simulink model "Rod_end_v7c"  (R2023a)
settings: Solver=ode1be  StartTime=0.0  StopTime=3  FixedStep=1e-6  MaxStep=1e-5  RelTol=1e-3
values from neighbouring files (symbols this model uses):
  A1_la = 5.710000e-003    (= 0.00571)    [C1_Actuator_1_Data.m]
  A2_la = 5.710000e-003    (= 0.00571)    [C1_Actuator_1_Data.m]
  a_jetpipe_area = 0    [B2_Main_file_Double_Active_Standby_System.m]
  A_svfb = 79.12.*1E-9.*sqrt(pi)    [B2_Main_file_Double_Active_Standby_System.m]
  a_svfb0_1 = 1E-3    (= 0.001)    [B2_Main_file_Double_Active_Standby_System.m]
  a_svfb0_2 = 0    [B2_Main_file_Double_Active_Standby_System.m]
  Afl_sv = dfl_sv^2*pi/4    (= 2.01519637574e-09)    [C1_Actuator_1_Data.m]
  Ag_sv = 18e-6    (= 1.8e-05)    [C1_Actuator_1_Data.m]
  air_gap0_1 = 0    [B2_Main_file_Double_Active_Standby_System.m]
  air_gap_fault_time = 10000    [B2_Main_file_Double_Active_Standby_System.m]
  Alpha_p0 = eta-acos((L^2+t^2-s^2)/(2*L*t))    [Parametri_rod_end.m]
  Asp_sv = 1.35e-5    (= 1.35e-05)    [C1_Actuator_1_Data.m]
  B0_sv = 0.460    (= 0.46)    [C1_Actuator_1_Data.m]
  b_airgap = 0.3    [B2_Main_file_Double_Active_Standby_System.m]
  b_fbspring = 2E-3    (= 0.002)    [B2_Main_file_Double_Active_Standby_System.m]
  b_max = 0*0.0001    (= 0)    [C1_Actuator_1_Data.m]
  beta = 800000000    [D4_Fluid.m]    (also in Rapporto_di_trasmissione.m = acos((L-t.*cos(alpha))./s))
  Beta0 = acos((L-t*cos(Alpha0))/s)    [Parametri_rod_end.m]
  beta_LVDT = 0    [aggiunte.m]
  bf_sv = 0.45    [C1_Actuator_1_Data.m]
  bsp_sv = 0.25    [C1_Actuator_1_Data.m]
  c = 55    [Parametri_rod_end.m]
  C_svfb = 1    [B2_Main_file_Double_Active_Standby_System.m]
  Cdmax_sv = 0.7392    [C1_Actuator_1_Data.m]
  Cdmin_sv = 0.6428    [C1_Actuator_1_Data.m]
  CLa = 900000    [aggiunte.m]
  Csa_la = 0.02*sqrt(Ksa_la*Meq_la)    [C1_Actuator_1_Data.m]
  Damping = 1e3    (= 1000)    [Parametri_rod_end.m]
  Damping_rot = 100    [Parametri_rod_end.m]
  Del_on = 1    [B2_Main_file_Double_Active_Standby_System.m]
  demag0_1 = 0    [B2_Main_file_Double_Active_Standby_System.m]
  dfl_sv = 5.0654e-5    (= 5.0654e-05)    [C1_Actuator_1_Data.m]
  dt_sim = 1e-5    (= 1e-05)    [B2_Main_file_Double_Active_Standby_System.m]
  enable_jetpipe_distorsion = 0    [B2_Main_file_Double_Active_Standby_System.m]
  eta = deg2rad(15)    [Parametri_rod_end.m]
  F_att_sv = 4    [C1_Actuator_1_Data.m]
  FH = FH+0.175*pi*Dd_se(ii)*(-0.884+0.0206*Hs_se(ii)-0.0001*(Hs_se(ii))^2)*Tw_se(ii)    [D2_Data_seal.m]
  first_cycle = 0    [B2_Main_file_Double_Active_Standby_System.m]
  flight_hours = 8    [B2_Main_file_Double_Active_Standby_System.m]
  g = 9.81    [Parametri_rod_end.m]
  g_sv = G_sv/l0_sv    (= 0)    [C1_Actuator_1_Data.m]
  Gamma_la = 1.667e4    (= 16670)    [C1_Actuator_1_Data.m]
  gap_ms = 0    [C1_Actuator_1_Data.m]
  Gq_sv = 0.069    [C1_Actuator_1_Data.m]
  Gust_stiffness_jetpipe = 1e8    (= 100000000)    [B2_Main_file_Double_Active_Standby_System.m]
  Gust_threshold = 10000    [B2_Main_file_Double_Active_Standby_System.m]
  h_fbspring = 1E-3    (= 0.001)    [B2_Main_file_Double_Active_Standby_System.m]
  h_sv = H_sv/l0_sv    (= 0)    [C1_Actuator_1_Data.m]
  hr_sv = 6e-6    (= 6e-06)    [C1_Actuator_1_Data.m]
  hyd_fluid_repl = 20    [B2_Main_file_Double_Active_Standby_System.m]
  I = 2.3    [Parametri_rod_end.m]    (also in Rapporto_di_trasmissione.m)
  imax_sv = 8e-3    (= 0.008)    [C1_Actuator_1_Data.m]
  Initial_condition = [0;0;0.000]    [Parametri_rod_end.m]
  Ixx_out = 0.0000321    (= 3.21e-05)    [Parametri_rod_end.m]
  Iyy_in = 0.0000008    (= 8e-07)    [Parametri_rod_end.m]
  Iyy_out = 0.0000035    (= 3.5e-06)    [Parametri_rod_end.m]
  Izz_in = 0.00000011    (= 1.1e-07)    [Parametri_rod_end.m]
  Izz_out = 0.0000337    (= 3.37e-05)    [Parametri_rod_end.m]
  Ja_sv = 1.0575e-5    (= 1.0575e-05)    [C1_Actuator_1_Data.m]
  jetpipe_initialpos = 0    [B2_Main_file_Double_Active_Standby_System.m]
  jetpipe_passage_area = 1    [B2_Main_file_Double_Active_Standby_System.m]
  k = 4/(3*pi*(sigma_j+sigma_k))*((R_in*R_out)/(R_in+R_out))^0.5    (= 15092124693.8)    [Parametri_rod_end.m]
  k_airgap = 0.5/100*0.01    (= 5e-05)    [B2_Main_file_Double_Active_Standby_System.m]
  k_c0_jetpipe_area = 0*1e-1    (= 0)    [B2_Main_file_Double_Active_Standby_System.m]
  k_sv = mup_sv*Vp_sv/(2*B0_sv*l0_sv)-1    (= 16.0383594613)    [C1_Actuator_1_Data.m]
  Kf_sv = 301.6    [C1_Actuator_1_Data.m]
  KFPi = zeros(m,1)    [D2_Data_seal.m]
  Kli1 = 0    [C1_Actuator_1_Data.m]
  Kli2 = 0    [C1_Actuator_1_Data.m]
  Ksa_la = 12480000    [C1_Actuator_1_Data.m]
  Kw_sv = 14.5    [C1_Actuator_1_Data.m]
  L = 0.37    [Parametri_rod_end.m]    (also in Rapporto_di_trasmissione.m = l+delta_l)
  l0_sv = 0.5e-3    (= 0.0005)    [C1_Actuator_1_Data.m]
  L_c = imax_sv    (= 0.008)    [C1_Actuator_1_Data.m]
  L_la1 = 0.059900    (= 0.0599)    [C1_Actuator_1_Data.m]
  L_la2 = 0.084800    (= 0.0848)    [C1_Actuator_1_Data.m]
  la_sv = 41e-3    (= 0.041)    [C1_Actuator_1_Data.m]
  lambda_LVDT = 0*0.005*1.5    (= 0)    [aggiunte.m]
  lf = 0.025    [C1_Actuator_1_Data.m]    (also in C2_Actuator_2_Data.m)
  LVDTsize0 = 1    [aggiunte.m]
  m_in = 0.0215    [Parametri_rod_end.m]
  m_out = 0.1    [Parametri_rod_end.m]
  m_thermal = 0    [B2_Main_file_Double_Active_Standby_System.m]
  Mcyl_la = 30.425550    (= 30.42555)    [C1_Actuator_1_Data.m]
  Mrod_la = 11.313490    (= 11.31349)    [C1_Actuator_1_Data.m]
  msp_sv = 0.005    [C1_Actuator_1_Data.m]
  mua_sv = 4*pi/1e7    (= 1.25663706144e-06)    [C1_Actuator_1_Data.m]
  mup_sv = 1.1*4*pi/1e7    (= 1.38230076758e-06)    [C1_Actuator_1_Data.m]
  n1_sv = 1140    [C1_Actuator_1_Data.m]
  n2_sv = 1140    [C1_Actuator_1_Data.m]
  n_svfb = 3    [B2_Main_file_Double_Active_Standby_System.m]
  null_shift = -1+2*rand(1,1)    [B2_Main_file_Double_Active_Standby_System.m]
  null_shift_sign = -1+((-1+2*rand(1,1))>=0)*2    [B2_Main_file_Double_Active_Standby_System.m]
  OV_R1 = 0*2.344e-05    (= 0)    [C1_Actuator_1_Data.m]
  OV_R2 = 0*2.344e-05    (= 0)    [C1_Actuator_1_Data.m]
  OV_S1 = 0*2.344e-05    (= 0)    [C1_Actuator_1_Data.m]
  OV_S2 = 0*2.344e-05    (= 0)    [C1_Actuator_1_Data.m]
  P01_la = Pmean-DP_eq    [C1_Actuator_1_Data.m]
  P02_la = Pmean+DP_eq    [C1_Actuator_1_Data.m]
  perc_passage_area0_1 = 0    [B2_Main_file_Double_Active_Standby_System.m]
  Pocl_A = 0    [C1_Actuator_1_Data.m]
  Pocl_B = 0    [C1_Actuator_1_Data.m]
  Pr = 600000    [B2_Main_file_Double_Active_Standby_System.m]
  Ps = 35000000    [B2_Main_file_Double_Active_Standby_System.m]
  R_in = 0.019    [Parametri_rod_end.m]
  R_out = 0.0195    [Parametri_rod_end.m]
  R_th1 = 0    [B2_Main_file_Double_Active_Standby_System.m]
  Remax_sv = 5000    [C1_Actuator_1_Data.m]
  Resistance = 1    [C1_Actuator_1_Data.m]
  rj_sv = 1e-6    (= 1e-06)    [C1_Actuator_1_Data.m]
  Rp02_svspring = 1014    [B2_Main_file_Double_Active_Standby_System.m]
  s = 0.11    [Parametri_rod_end.m]    (also in Rapporto_di_trasmissione.m)
  sigma_0LVDT = 0*0.01*1.5*5    (= 0)    [aggiunte.m]
  ST_AD = ceil(10000/fs_AD)/10000    [C1_Actuator_1_Data.m]
  Stiffness_rot = 1e3    (= 1000)    [Parametri_rod_end.m]
  Stifness = 1e8    (= 100000000)    [Parametri_rod_end.m]
  sv_crackON1 = 0    [B2_Main_file_Double_Active_Standby_System.m]
  sv_crackON2 = 0    [B2_Main_file_Double_Active_Standby_System.m]
  T0 = 0    [aggiunte.m]
  tau_w1 = 0    [B2_Main_file_Double_Active_Standby_System.m]
  ... (+14 more)
undefined symbols (not defined in the file or in its folder): Ixx_in, magnitude, mass, muu, Newton, R_sp_C, Raphson
libraries: simulink x16, matrix_library x12, sharedutil x2
(part 1 of 4)
settings Model: SimulationMode=accelerator  Creator=ciro1  LastModifiedBy=ciro1
settings SolverCC: ODENIntegrationMethod=ode1be

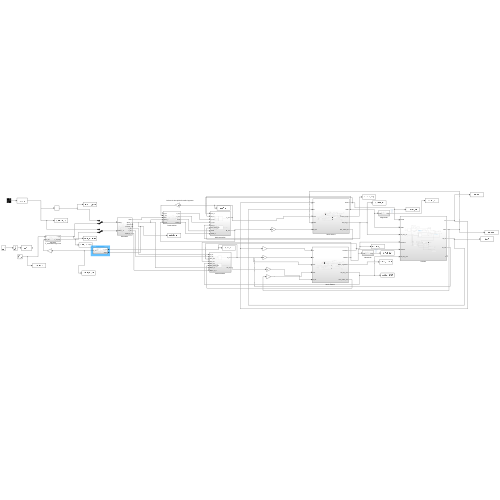
[thumbnail: Simulink's stored preview of the top-level diagram]
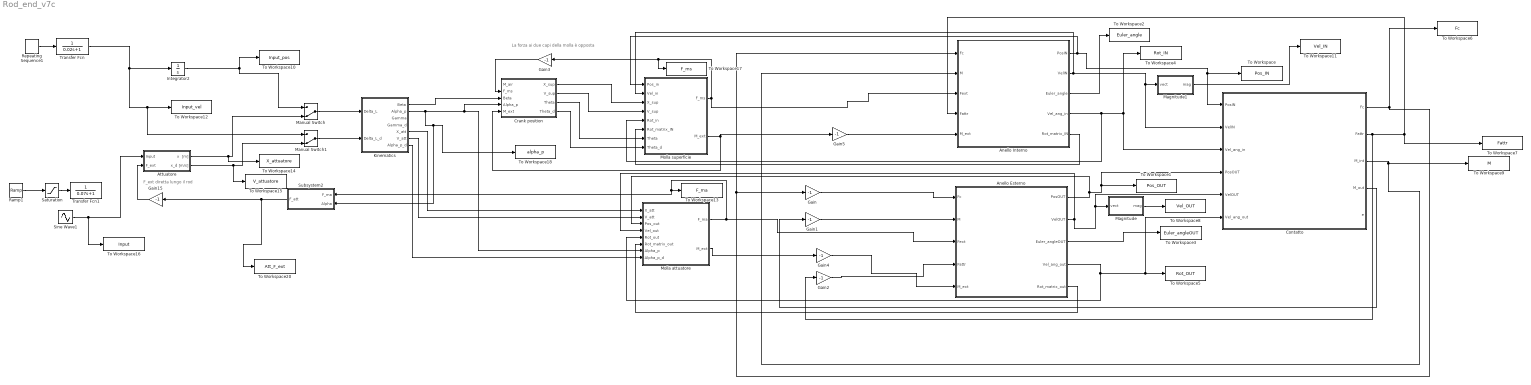
== system Rod_end_v7c ==
  note: F_ext diretta lungo il rod
  note: La forza ai due capi della molla è opposta
  Anello Esterno : Subsystem
  Anello Interno : Subsystem
  Attuatore : Subsystem
  Contatto : Subsystem
  Crank position : Subsystem
  Gain{,1..5,15} (7 alike) : Gain  Gain=-1
  Integrator2 : Integrator
  Kinematics : Subsystem
  Magnitude : Subsystem
  Magnitude1 : Subsystem
  Manual Switch : ManualSwitch  CurrentSetting=0
  Manual Switch1 : ManualSwitch  CurrentSetting=0
  Molla attuatore : Subsystem
  Molla superficie : Subsystem
  Ramp1 : simulink/Sources/Ramp  slope=0.035  start=0.2  InitialOutput=0
  Repeating Sequence1 : simulink/Sources/Repeating Sequence  rep_seq_t=[0 0.33 0.66 1 1.33 1.66 2]  rep_seq_y=[0 0.05 0.05 0 -0.05 -0.05 0]
  Saturation : Saturate  UpperLimit=0.045
  Sine Wave1 : Sin  Amplitude=0.05  Frequency=3.5  SampleTime=0
  Subsystem2 : Subsystem
  To Workspace : ToWorkspace  VariableName=Pos_IN  SampleTime=-1
  To Workspace1 : ToWorkspace  VariableName=Pos_OUT  SampleTime=-1
  To Workspace10 : ToWorkspace  VariableName=Input_pos  SampleTime=-1
  To Workspace11 : ToWorkspace  VariableName=Vel_IN  SampleTime=-1
  To Workspace12 : ToWorkspace  VariableName=Input_vel  SampleTime=-1
  To Workspace13 : ToWorkspace  VariableName=F_ma  SampleTime=-1
  To Workspace14 : ToWorkspace  VariableName=X_attuatore  SampleTime=-1
  To Workspace15 : ToWorkspace  VariableName=V_attuatore  SampleTime=-1
  To Workspace16 : ToWorkspace  VariableName=Input  SampleTime=-1
  To Workspace17 : ToWorkspace  VariableName=F_ms  SampleTime=-1
  To Workspace18 : ToWorkspace  VariableName=alpha_p  SampleTime=-1
  To Workspace2 : ToWorkspace  VariableName=Euler_angle  SampleTime=-1
  To Workspace20 : ToWorkspace  VariableName=Att_F_ext  SampleTime=-1
  To Workspace3 : ToWorkspace  VariableName=Euler_angleOUT  SampleTime=-1
  To Workspace4 : ToWorkspace  VariableName=Rot_IN  SampleTime=-1
  To Workspace5 : ToWorkspace  VariableName=Rot_OUT  SampleTime=-1
  To Workspace6 : ToWorkspace  VariableName=Fc  SampleTime=-1
  To Workspace7 : ToWorkspace  VariableName=Fattr  SampleTime=-1
  To Workspace8 : ToWorkspace  VariableName=Vel_OUT  SampleTime=-1
  To Workspace9 : ToWorkspace  VariableName=M  SampleTime=-1
  Transfer Fcn : TransferFcn  Denominator=[0.02 1]
  Transfer Fcn1 : TransferFcn  Denominator=[0.07 1]
  wires:
  Anello Esterno/2(VelOUT) -> Molla attuatore/4(Vel_out), Magnitude/1(vect), Contatto/5(VelOUT)
  Anello Esterno/3(Euler_angleOUT) -> To Workspace3/1
  Contatto/1(Fc) -> To Workspace6/1, Gain/1, Anello Interno/1(Fc)
  Contatto/4(M_out) -> Gain1/1
  Anello Interno/2(VelIN) -> Magnitude1/1(vect), Contatto/2(VelIN), Molla superficie/2(Vel_in)
  Anello Esterno/1(PosOUT) -> Molla attuatore/3(Pos_out), Contatto/4(PosOUT), To Workspace1/1
  Kinematics/5(X_att) -> Molla attuatore/1(X_att)
  Kinematics/1(Beta) -> Crank position/3(Beta)
  Kinematics/2(Alpha_p) -> Subsystem2/2(Alpha), To Workspace18/1, Molla attuatore/7(Alpha_p), Crank position/4(Alpha_p)
  Crank position/2(V_sup) -> Molla superficie/4(V_sup)
  Gain/1 -> Anello Esterno/1(Fc)
  Anello Esterno/5(Rot_matrix_out) -> Molla attuatore/6(Rot_matrix_out)
  Anello Interno/3(Euler_angle) -> To Workspace2/1
  Anello Interno/5(Rot_matrix_IN) -> Molla superficie/6(Rot_matrix_IN)
  Kinematics/6(V_att) -> Molla attuatore/2(V_att)
  Gain3/1 -> Crank position/2(F_ms)
  Molla attuatore/2(M_ext) -> Gain4/1
  Molla attuatore/1(F_ma) -> Anello Esterno/3(Fext), Subsystem2/1(F_ma), To Workspace13/1
  Gain4/1 -> Anello Esterno/5(M_ext)
  Molla superficie/1(F_ms) -> Anello Interno/3(Fext), To Workspace17/1, Gain3/1
  Gain5/1 -> Anello Interno/5(M_ext)
  Anello Interno/1(PosIN) -> Molla superficie/1(Pos_in), To Workspace/1, Contatto/1(PosIN)
  Crank position/1(X_sup) -> Molla superficie/3(X_sup)
  Anello Esterno/4(Vel_ang_out) -> Molla attuatore/5(Rot_out), To Workspace5/1, Contatto/6(Vel_ang_out)
  Gain2/1 -> Anello Esterno/4(Fattr)
  Gain1/1 -> Anello Esterno/2(M)
  Contatto/3(M_int) -> Anello Interno/2(M), To Workspace9/1
  Contatto/2(Fattr) -> Gain2/1, Anello Interno/4(Fattr), To Workspace7/1
  Anello Interno/4(Vel_ang_in) -> Molla superficie/5(Rot_in), Contatto/3(Vel_ang_in), To Workspace4/1
  Integrator2/1 -> To Workspace10/1, Manual Switch/1
  Crank position/3(Theta) -> Molla superficie/7(Theta)
  Magnitude/1(mag) -> To Workspace8/1
  Magnitude1/1(mag) -> To Workspace11/1
  Crank position/4(Theta_d) -> Molla superficie/8(Theta_d)
  Kinematics/7(Alpha_p_d) -> Molla attuatore/8(Alpha_p_d)
  Manual Switch/1 -> Kinematics/1(Delta_L)
  Manual Switch1/1 -> Kinematics/2(Delta_L_d)
  Attuatore/2(x_d [m/s]) -> To Workspace15/1, Manual Switch1/2
  Subsystem2/1(F_att) -> To Workspace20/1, Gain15/1
  Attuatore/1(x  [m]) -> To Workspace14/1, Manual Switch/2
  Saturation/1 -> Transfer Fcn1/1
  Ramp1/1 -> Saturation/1
  Gain15/1 -> Attuatore/2(F_ext)
  Sine Wave1/1 -> To Workspace16/1, Attuatore/1(Input)
  Molla superficie/2(M_ext) -> Crank position/5(M_ext), Gain5/1
  Repeating Sequence1/1 -> Transfer Fcn/1
  Transfer Fcn/1 -> Manual Switch1/1, To Workspace12/1, Integrator2/1

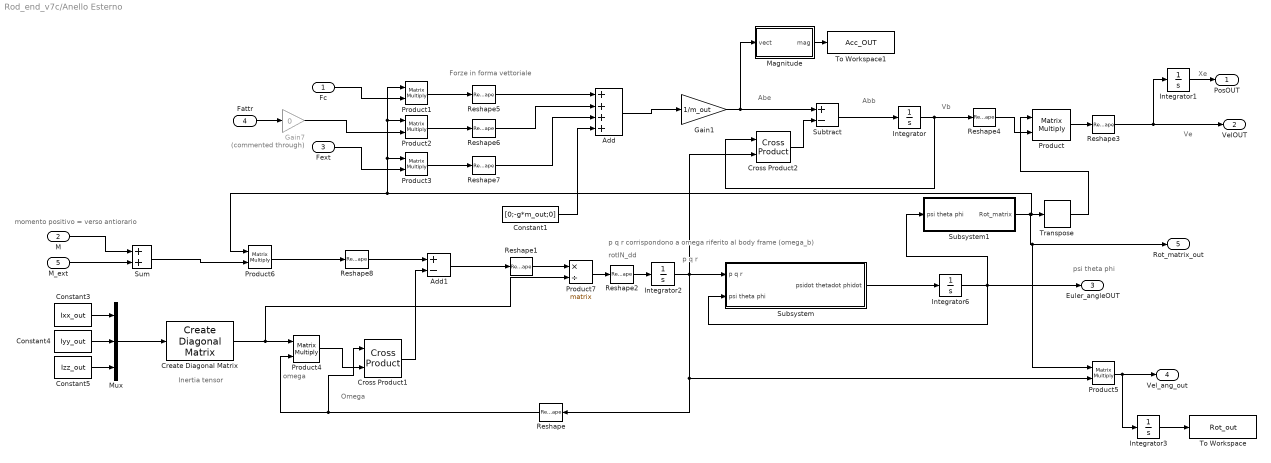
== system Rod_end_v7c/Anello Esterno ==
  note: momento positivo = verso antiorario
  note: Xe
  note: Ve
  note: Vb
  note: Abb
  note: p q r corrispondono a omega riferito al body frame (omega_b)
  note: psi theta phi
  note: p q r
  note: Omega
  note: omega
  note: Forze in forma vettoriale
  note: Abe
  note: Inertia tensor
  note: rotIN_dd
  Fc : Inport
  M : Inport  Port=2
  Fext : Inport  Port=3
  Fattr : Inport  Port=4
  M_ext : Inport  Port=5
  Add : Sum  Inputs=++++
  Add1 : Sum  Inputs=+-
  Constant1 : Constant  Value=[0;-g*m_out;0]
  Constant3 : Constant  Value=Ixx_out
  Constant4 : Constant  Value=Iyy_out
  Constant5 : Constant  Value=Izz_out
  Create Diagonal Matrix : matrix_library/Create Diagonal Matrix
      settings: LibrarySourceBlock=|
      | simulink/Matrix
      | Operations/Create Diagonal
      | Matrix
  Cross Product1 : matrix_library/Cross Product
  Cross Product2 : matrix_library/Cross Product
  Gain1 : Gain  Gain=1/m_out
  Gain7 : Gain  Commented=through  Gain=0
  Integrator : Integrator
  Integrator1 : Integrator  InitialCondition=Initial_condition
  Integrator2 : Integrator
  Integrator3 : Integrator
  Integrator6 : Integrator  WrapState=on
  Magnitude : Subsystem
  Mux : Mux  Inputs=3
  Product{,1..3,5..6} (6 alike) : Product  Multiplication=Matrix(*)
  Product4 : Product  Inputs=**  Multiplication=Matrix(*)
  Product7 : Product  Inputs=*/  Multiplication=Matrix(*)
  Reshape : Reshape  OutputDimensionality=Column vector (2-D)
  Reshape1 : Reshape  OutputDimensionality=Row vector (2-D)
  Reshape{2..3,5..8} (6 alike) : Reshape
  Reshape4 : Reshape  OutputDimensionality=Column vector (2-D)
  Subsystem : Subsystem
  Subsystem1 : Subsystem
  Subtract : Sum  Inputs=+-
  Sum : Sum
  To Workspace : ToWorkspace  VariableName=Rot_out  SampleTime=-1
  To Workspace1 : ToWorkspace  VariableName=Acc_OUT  SampleTime=-1
  Transpose : matrix_library/Transpose
  PosOUT : Outport
  VelOUT : Outport  Port=2
  Euler_angleOUT : Outport  Port=3
  Vel_ang_out : Outport  Port=4
  Rot_matrix_out : Outport  Port=5
  wires:
  Gain1/1 -> Magnitude/1(vect), Subtract/1
  Constant3/1 -> Mux/1
  Constant4/1 -> Mux/2
  Mux/1 -> Create Diagonal Matrix/1
  Constant5/1 -> Mux/3
  Cross Product1/1 -> Add1/2
  Product7/1 -> Reshape2/1
  Add1/1 -> Reshape1/1
  Reshape1/1 -> Product7/1
  Subsystem/1(psidot thetadot phidot) -> Integrator6/1
  Reshape2/1 -> Integrator2/1
  Subtract/1 -> Integrator/1
  Integrator/1 -> Cross Product2/1, Reshape4/1
  Cross Product2/1 -> Subtract/2
  Subsystem1/1(Rot_matrix) -> Rot_matrix_out/1, Product5/1, Product6/1, Product3/1, Product2/1, Product1/1, Transpose/1
  Product/1 -> Reshape3/1
  Integrator1/1 -> PosOUT/1
  Reshape3/1 -> Integrator1/1, VelOUT/1
  Integrator6/1 -> Euler_angleOUT/1, Subsystem/2(psi theta phi), Subsystem1/1(psi theta phi)
  Reshape4/1 -> Product/2
  Transpose/1 -> Product/1
  Product4/1 -> Cross Product1/2
  Reshape/1 -> Cross Product1/1, Product4/2
  Product1/1 -> Reshape5/1
  Fc/1 -> Product1/2
  Fattr/1 -> Gain7/1
  Fext/1 -> Product3/2
  Product2/1 -> Reshape6/1
  Reshape6/1 -> Add/2
  Product3/1 -> Reshape7/1
  Reshape7/1 -> Add/3
  Reshape8/1 -> Add1/1
  Reshape5/1 -> Add/1
  M_ext/1 -> Sum/2
  M/1 -> Sum/1
  Constant1/1 -> Add/4
  Gain7/1 -> Product2/2
  Integrator3/1 -> To Workspace/1
  Product5/1 -> Integrator3/1, Vel_ang_out/1
  Magnitude/1(mag) -> To Workspace1/1
  Product6/1 -> Reshape8/1
  Add/1 -> Gain1/1
  Integrator2/1 -> Product5/2, Reshape/1, Cross Product2/2, Subsystem/1(p q r)
  Create Diagonal Matrix/1 -> Product7/2, Product4/1
  Sum/1 -> Product6/2

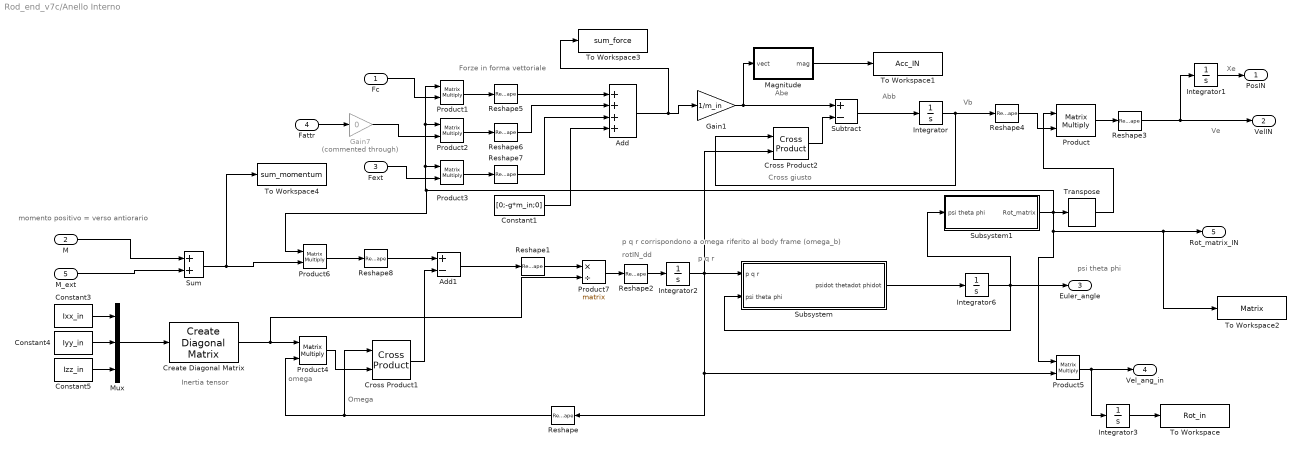
== system Rod_end_v7c/Anello Interno ==
  note: momento positivo = verso antiorario
  note: Cross giusto
  note: Xe
  note: Ve
  note: Vb
  note: Abb
  note: p q r corrispondono a omega riferito al body frame (omega_b)
  note: psi theta phi
  note: p q r
  note: Omega
  note: omega
  note: Forze in forma vettoriale
  note: Abe
  note: Inertia tensor
  note: rotIN_dd
  Fc : Inport
  M : Inport  Port=2
  Fext : Inport  Port=3
  Fattr : Inport  Port=4
  M_ext : Inport  Port=5
  Add : Sum  Inputs=++++
  Add1 : Sum  Inputs=+-
  Constant1 : Constant  Value=[0;-g*m_in;0]
  Constant3 : Constant  Value=Ixx_in
  Constant4 : Constant  Value=Iyy_in
  Constant5 : Constant  Value=Izz_in
  Create Diagonal Matrix : matrix_library/Create Diagonal Matrix
      settings: LibrarySourceBlock=|
      | simulink/Matrix
      | Operations/Create Diagonal
      | Matrix
  Cross Product1 : matrix_library/Cross Product
  Cross Product2 : matrix_library/Cross Product
  Gain1 : Gain  Gain=1/m_in
  Gain7 : Gain  Commented=through  Gain=0
  Integrator{,1..3} (4 alike) : Integrator
  Integrator6 : Integrator  WrapState=on
  Magnitude : Subsystem
  Mux : Mux  Inputs=3
  Product{,1..3,5..6} (6 alike) : Product  Multiplication=Matrix(*)
  Product4 : Product  Inputs=**  Multiplication=Matrix(*)
  Product7 : Product  Inputs=*/  Multiplication=Matrix(*)
  Reshape : Reshape  OutputDimensionality=Column vector (2-D)
  Reshape1 : Reshape  OutputDimensionality=Row vector (2-D)
  Reshape{2..3,5..8} (6 alike) : Reshape
  Reshape4 : Reshape  OutputDimensionality=Column vector (2-D)
  Subsystem : Subsystem
  Subsystem1 : Subsystem
  Subtract : Sum  Inputs=+-
  Sum : Sum
  To Workspace : ToWorkspace  VariableName=Rot_in  SampleTime=-1
  To Workspace1 : ToWorkspace  VariableName=Acc_IN  SampleTime=-1
  To Workspace2 : ToWorkspace  VariableName=Matrix  SaveFormat=Timeseries  SampleTime=-1
  To Workspace3 : ToWorkspace  VariableName=sum_force  SampleTime=-1
  To Workspace4 : ToWorkspace  VariableName=sum_momentum  SampleTime=-1
  Transpose : matrix_library/Transpose
  PosIN : Outport
  VelIN : Outport  Port=2
  Euler_angle : Outport  Port=3
  Vel_ang_in : Outport  Port=4
  Rot_matrix_IN : Outport  Port=5
  wires:
  Add/1 -> To Workspace3/1, Gain1/1
  Constant3/1 -> Mux/1
  Constant4/1 -> Mux/2
  Mux/1 -> Create Diagonal Matrix/1
  Create Diagonal Matrix/1 -> Product4/1, Product7/2
  Constant5/1 -> Mux/3
  Cross Product1/1 -> Add1/2
  Product7/1 -> Reshape2/1
  Reshape/1 -> Cross Product1/1, Product4/2
  Add1/1 -> Reshape1/1
  Reshape1/1 -> Product7/1
  Integrator2/1 -> Product5/2, Reshape/1, Cross Product2/2, Subsystem/1(p q r)
  Subsystem/1(psidot thetadot phidot) -> Integrator6/1
  Reshape2/1 -> Integrator2/1
  Integrator/1 -> Cross Product2/1, Reshape4/1
  Cross Product2/1 -> Subtract/2
  Product/1 -> Reshape3/1
  Integrator1/1 -> PosIN/1
  Reshape3/1 -> Integrator1/1, VelIN/1
  Integrator6/1 -> Euler_angle/1, Subsystem/2(psi theta phi), Subsystem1/1(psi theta phi)
  Reshape4/1 -> Product/2
  Transpose/1 -> Product/1
  Constant1/1 -> Add/4
  Subtract/1 -> Integrator/1
  Product4/1 -> Cross Product1/2
  Gain1/1 -> Subtract/1, Magnitude/1(vect)
  Product1/1 -> Reshape5/1
  Fc/1 -> Product1/2
  Reshape5/1 -> Add/1
  Fattr/1 -> Gain7/1
  Fext/1 -> Product3/2
  Product3/1 -> Reshape7/1
  Product2/1 -> Reshape6/1
  Reshape7/1 -> Add/3
  Reshape6/1 -> Add/2
  Product5/1 -> Integrator3/1, Vel_ang_in/1
  Reshape8/1 -> Add1/1
  Product6/1 -> Reshape8/1
  M/1 -> Sum/1
  M_ext/1 -> Sum/2
  Sum/1 -> To Workspace4/1, Product6/2
  Gain7/1 -> Product2/2
  Integrator3/1 -> To Workspace/1
  Magnitude/1(mag) -> To Workspace1/1
  Subsystem1/1(Rot_matrix) -> To Workspace2/1, Rot_matrix_IN/1, Product5/1, Product6/1, Product3/1, Product2/1, Product1/1, Transpose/1

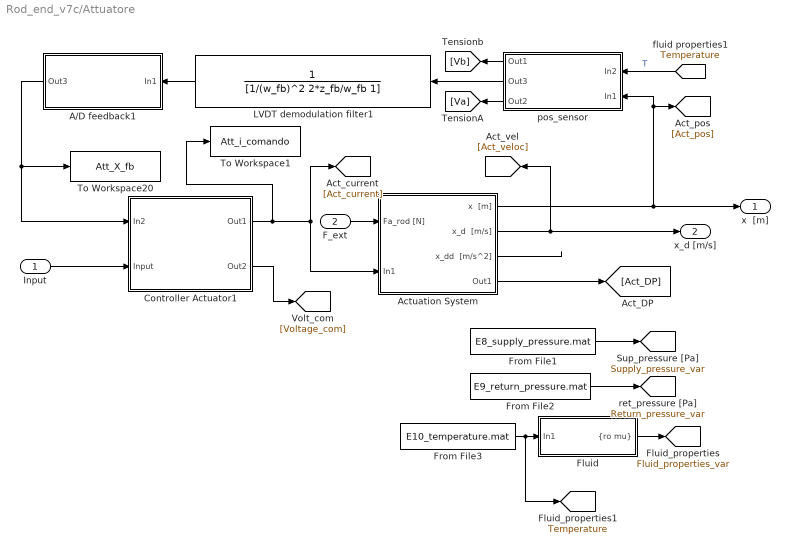
== system Rod_end_v7c/Attuatore ==
  Input : Inport
  F_ext : Inport  Port=2
  A/D feedback1 : Subsystem
  Actuation System : Subsystem
  Controller Actuator1 : Subsystem
  Fluid : Subsystem
  From File1 : FromFile  FileName=E8_supply_pressure.mat  SampleTime=dt_sim
  From File2 : FromFile  FileName=E9_return_pressure.mat  SampleTime=dt_sim
  From File3 : FromFile  FileName=E10_temperature.mat  SampleTime=dt_sim
  LVDT demodulation filter1 : TransferFcn  Denominator=[1/(w_fb)^2 2*z_fb/w_fb 1]
  To Workspace1 : ToWorkspace  VariableName=Att_i_comando  SampleTime=-1
  To Workspace20 : ToWorkspace  VariableName=Att_X_fb  SampleTime=-1
  pos_sensor : Subsystem
  x  [m] : Outport
  x_d [m/s] : Outport  Port=2
  tag scope: Fluid_properties_var=global, Return_pressure_var=global, Supply_pressure_var=global, Temperature=global
  wires:
  A/D feedback1/1(Out3) -> To Workspace20/1, Controller Actuator1/1(In2)
  pos_sensor/1(Out1) -> [Vb]
  pos_sensor/3(Out2) -> [Va]
  Actuation System/1(x  [m]) -> pos_sensor/2(In1), [Act_pos], x  [m]/1
  From File1/1 -> [Supply_pressure_var]
  From File2/1 -> [Return_pressure_var]
  Actuation System/2(x_d  [m/s]) -> [Act_veloc], x_d [m/s]/1
  LVDT demodulation filter1/1 -> A/D feedback1/1(In1)
  [Temperature] -> pos_sensor/1(In2)  "T"
  Actuation System/4(Out1) -> [Act_DP]
  Controller Actuator1/1(Out1) -> [Act_current], Actuation System/2(In1), To Workspace1/1
  Fluid/1("{ro mu}") -> [Fluid_properties_var]
  Actuation System/3(x_dd  [m/s^2]) -> ?
  From File3/1 -> [Temperature], Fluid/1(In1)
  Controller Actuator1/2(Out2) -> [Voltage_com]
  pos_sensor/2(Out3) -> LVDT demodulation filter1/1
  Input/1 -> Controller Actuator1/2(Input)
  F_ext/1 -> Actuation System/1(Fa_rod [N])

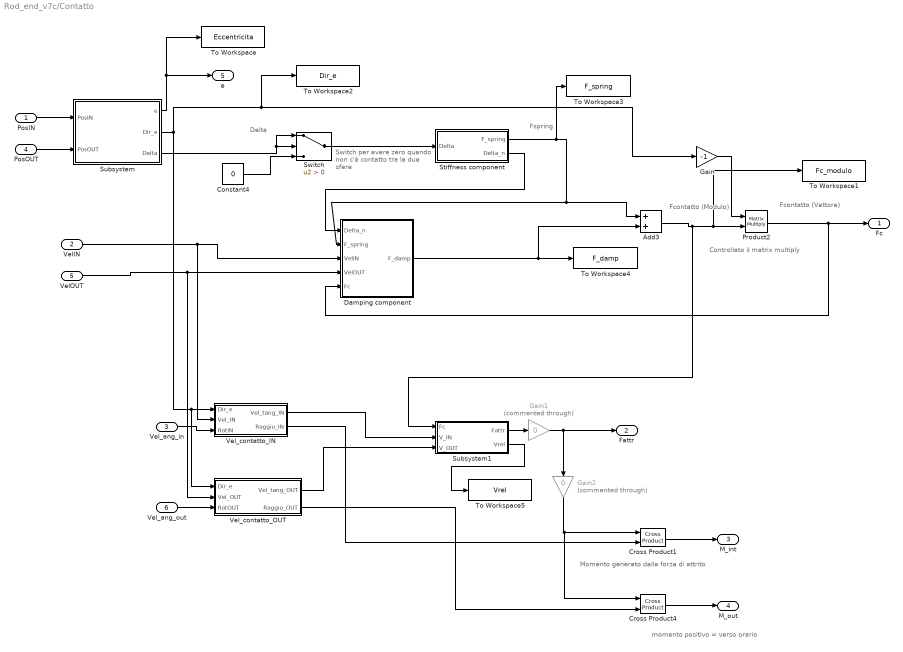
== system Rod_end_v7c/Contatto ==
  note: momento positivo = verso orario
  note: Controllato il matrix multiply
  note: Switch per avere zero quando non c'è contatto
      | tra le due sfere
  note: Momento generato dalla forza di attrito
  note: Fcontatto
      | (Vettore)
  note: Fcontatto
      | (Modulo)
  note: Fspring
  note: Delta
  PosIN : Inport
  VelIN : Inport  Port=2
  Vel_ang_in : Inport  Port=3
  PosOUT : Inport  Port=4
  VelOUT : Inport  Port=5
  Vel_ang_out : Inport  Port=6
  Add3 : Sum
  Constant4 : Constant  Value=0
  Cross Product1 : matrix_library/Cross Product
  Cross Product4 : matrix_library/Cross Product
  Damping component : Subsystem
  Gain : Gain  Gain=-1
  Gain1 : Gain  Commented=through  Gain=0
  Gain2 : Gain  Commented=through  Gain=0
  Product2 : Product  Multiplication=Matrix(*)
  Stiffness component : Subsystem
  Subsystem : Subsystem
  Subsystem1 : Subsystem
  Switch : Switch  Criteria=u2 > Threshold  SaturateOnIntegerOverflow=off  InputSameDT=off
  To Workspace : ToWorkspace  VariableName=Eccentricita  SampleTime=-1
  To Workspace1 : ToWorkspace  VariableName=Fc_modulo  SampleTime=-1
  To Workspace2 : ToWorkspace  VariableName=Dir_e  SampleTime=-1
  To Workspace3 : ToWorkspace  VariableName=F_spring  SampleTime=-1
  To Workspace4 : ToWorkspace  VariableName=F_damp  SampleTime=-1
  To Workspace5 : ToWorkspace  VariableName=Vrel  SampleTime=-1
  Vel_contatto_IN : Subsystem
  Vel_contatto_OUT : Subsystem
  Fc : Outport
  Fattr : Outport  Port=2
  M_int : Outport  Port=3
  M_out : Outport  Port=4
  e : Outport  Port=5
  wires:
  Damping component/1(F_damp) -> Add3/2, To Workspace4/1
  Gain/1 -> Product2/1
  Subsystem/2(Dir_e) -> To Workspace2/1, Gain/1, Vel_contatto_OUT/1(Dir_e), Vel_contatto_IN/1(Dir_e)
  Cross Product1/1 -> M_int/1
  Stiffness component/1(F_spring) -> To Workspace3/1, Damping component/2(F_spring), Add3/1
  Subsystem1/1(Fattr) -> Gain1/1
  Subsystem/3(Delta) -> Switch/2, Switch/1
  Constant4/1 -> Switch/3
  Add3/1 -> To Workspace1/1, Product2/2, Subsystem1/1(Fc)
  Cross Product4/1 -> M_out/1
  Product2/1 -> Damping component/5(Fc), Fc/1
  PosOUT/1 -> Subsystem/2(PosOUT)
  PosIN/1 -> Subsystem/1(PosIN)
  Switch/1 -> Stiffness component/1(Delta)
  Stiffness component/2(Delta_n) -> Damping component/1(Delta_n)
  Vel_ang_in/1 -> Vel_contatto_IN/3(RotIN)
  VelIN/1 -> Vel_contatto_IN/2(Vel_IN), Damping component/3(VelIN)
  Vel_ang_out/1 -> Vel_contatto_OUT/3(RotOUT)
  VelOUT/1 -> Damping component/4(VelOUT), Vel_contatto_OUT/2(Vel_OUT)
  Vel_contatto_IN/1(Vel_tang_IN) -> Subsystem1/2(V_IN)
  Vel_contatto_OUT/1(Vel_tang_OUT) -> Subsystem1/3(V_OUT)
  Vel_contatto_IN/2(Raggio_IN) -> Cross Product1/2
  Vel_contatto_OUT/2(Raggio_OUT) -> Cross Product4/2
  Subsystem/1(e) -> e/1, To Workspace/1
  Gain1/1 -> Fattr/1, Gain2/1
  Gain2/1 -> Cross Product1/1, Cross Product4/1
  Subsystem1/2(Vrel) -> To Workspace5/1

== system Rod_end_v7c/Crank position ==
  M_air : Inport
  F_ms : Inport  Port=2
  Beta : Inport  Port=3
  Alpha_p : Inport  Port=4
  M_ext : Inport  Port=5
  Moment : Subsystem
  Rot_equilibrium : Subsystem
  To Workspace : ToWorkspace  VariableName=Theta  SampleTime=-1
  Trigonometry for V_sup : Subsystem
  Trigonometry for x_sup : Subsystem
  X_sup : Outport
  V_sup : Outport  Port=2
  Theta : Outport  Port=3
  Theta_d : Outport  Port=4
  wires:
  Rot_equilibrium/1(Theta) -> To Workspace/1, Theta/1, Trigonometry for x_sup/1(Theta)
  Alpha_p/1 -> Moment/4(Alpha_p)
  F_ms/1 -> Moment/2(F_ms)
  Beta/1 -> Moment/3(Beta)
  Moment/1(M) -> Rot_equilibrium/1(M)
  Trigonometry for x_sup/1(X_sup) -> X_sup/1
  Trigonometry for V_sup/1(V_sup) -> V_sup/1
  Rot_equilibrium/2(Theta_d) -> Trigonometry for V_sup/1(Theta_d), Theta_d/1
  Trigonometry for x_sup/3(Cos_angle+theta) -> Trigonometry for V_sup/3(Cos)
  Trigonometry for x_sup/2(Sin_angle+theta) -> Rot_equilibrium/3(Angle), Trigonometry for V_sup/2(Sin)
  M_air/1 -> Moment/1(M_ext)
  M_ext/1 -> Rot_equilibrium/2(M_ext)

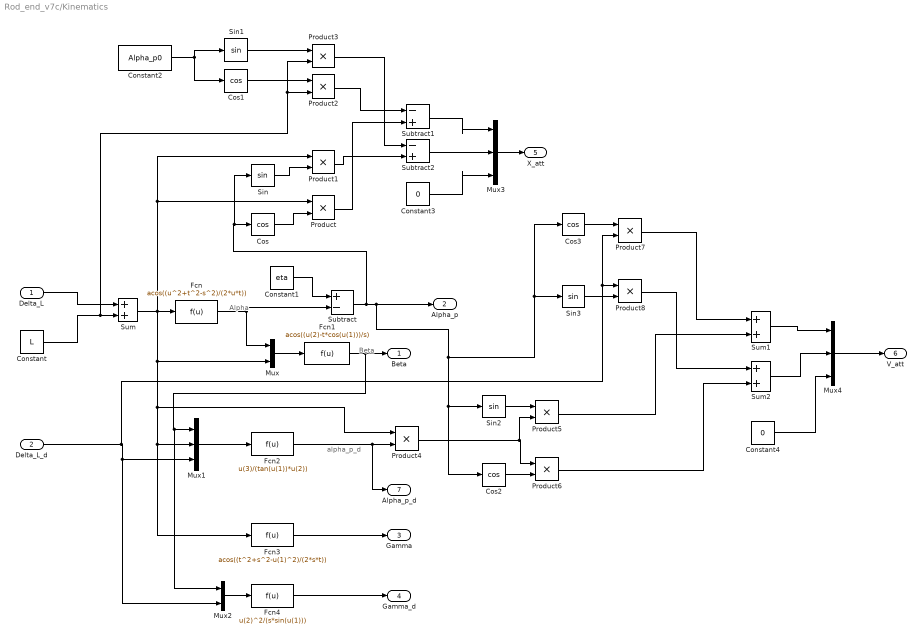
== system Rod_end_v7c/Kinematics ==
  note: alpha_p_d
  note: Beta
  note: Alpha
  Delta_L : Inport
  Delta_L_d : Inport  Port=2
  Constant : Constant  Value=L
  Constant1 : Constant  Value=eta
  Constant2 : Constant  Value=Alpha_p0
  Constant3 : Constant  Value=0
  Constant4 : Constant  Value=0
  Cos{,1..3} (4 alike) : Trigonometry  Operator=cos
  Fcn : Fcn  Expr=acos((u^2+t^2-s^2)/(2*u*t))
  Fcn1 : Fcn  Expr=acos((u(2)-t*cos(u(1)))/s)
  Fcn2 : Fcn  Expr=u(3)/(tan(u(1))*u(2))
  Fcn3 : Fcn  Expr=acos((t^2+s^2-u(1)^2)/(2*s*t))
  Fcn4 : Fcn  Expr=u(2)^2/(s*sin(u(1)))
  Mux : Mux  Inputs=2
  Mux1 : Mux  Inputs=3
  Mux2 : Mux  Inputs=2
  Mux3 : Mux  Inputs=3
  Mux4 : Mux  Inputs=3
  Product{,1..8} (9 alike) : Product
  Sin{,1..3} (4 alike) : Trigonometry
  Subtract : Sum  Inputs=+-
  Subtract1 : Sum  Inputs=-+
  Subtract2 : Sum  Inputs=-+
  Sum : Sum
  Sum1 : Sum
  Sum2 : Sum
  Beta : Outport
  Alpha_p : Outport  Port=2
  Gamma : Outport  Port=3
  Gamma_d : Outport  Port=4
  X_att : Outport  Port=5
  V_att : Outport  Port=6
  Alpha_p_d : Outport  Port=7
  wires:
  Constant/1 -> Product3/2, Product2/2, Sum/2
  Delta_L/1 -> Sum/1
  Sum/1 -> Product1/1, Product/1, Product4/1, Fcn3/1, Mux1/2, Mux/2, Fcn/1
  Fcn/1 -> Mux/1, Subtract/2
  Mux/1 -> Fcn1/1
  Constant1/1 -> Subtract/1
  Subtract/1 -> Sin/1, Cos/1, Cos2/1, Sin2/1, Cos3/1, Sin3/1, Alpha_p/1
  Mux1/1 -> Fcn2/1
  Fcn3/1 -> Gamma/1
  Mux2/1 -> Fcn4/1
  Fcn4/1 -> Gamma_d/1
  Sin/1 -> Product1/2
  Cos/1 -> Product/2
  Constant2/1 -> Cos1/1, Sin1/1
  Sin1/1 -> Product3/1
  Cos1/1 -> Product2/1
  Product1/1 -> Subtract2/2
  Product3/1 -> Subtract2/1
  Product2/1 -> Subtract1/1
  Product/1 -> Subtract1/2
  Subtract1/1 -> Mux3/1
  Constant3/1 -> Mux3/3
  Subtract2/1 -> Mux3/2
  Mux3/1 -> X_att/1
  Fcn2/1 -> Alpha_p_d/1, Product4/2
  Sin2/1 -> Product5/1
  Cos2/1 -> Product6/2
  Product4/1 -> Product5/2, Product6/1
  Product5/1 -> Sum1/2
  Product6/1 -> Sum2/2
  Cos3/1 -> Product7/1
  Sin3/1 -> Product8/2
  Product7/1 -> Sum1/1
  Product8/1 -> Sum2/1
  Sum1/1 -> Mux4/1
  Sum2/1 -> Mux4/2
  Constant4/1 -> Mux4/3
  Mux4/1 -> V_att/1
  Delta_L_d/1 -> Product8/1, Product7/2, Mux2/2, Mux1/3
  Fcn1/1 -> Mux2/1, Mux1/1, Beta/1

== system Rod_end_v7c/Magnitude ==
  vect : Inport
  Add2 : Sum  Inputs=+++
  Demux : Demux  Outputs=3
  Math Function : Math  Operator=square  SignedPower=on
  Math Function1 : Math  Operator=square  SignedPower=on
  Math Function2 : Math  Operator=square  SignedPower=on
  Sqrt : Sqrt
  mag : Outport  VectorParamsAs1DForOutWhenUnconnected=off
  wires:
  vect/1 -> Demux/1
  Add2/1 -> Sqrt/1
  Math Function2/1 -> Add2/3
  Demux/1 -> Math Function/1
  Math Function1/1 -> Add2/2
  Math Function/1 -> Add2/1
  Demux/3 -> Math Function2/1
  Demux/2 -> Math Function1/1
  Sqrt/1 -> mag/1

== system Rod_end_v7c/Magnitude1 ==
  vect : Inport
  Add2 : Sum  Inputs=+++
  Demux : Demux  Outputs=3
  Math Function : Math  Operator=square  SignedPower=on
  Math Function1 : Math  Operator=square  SignedPower=on
  Math Function2 : Math  Operator=square  SignedPower=on
  Sqrt : Sqrt
  mag : Outport  VectorParamsAs1DForOutWhenUnconnected=off
  wires:
  vect/1 -> Demux/1
  Add2/1 -> Sqrt/1
  Math Function2/1 -> Add2/3
  Demux/1 -> Math Function/1
  Math Function1/1 -> Add2/2
  Math Function/1 -> Add2/1
  Demux/3 -> Math Function2/1
  Demux/2 -> Math Function1/1
  Sqrt/1 -> mag/1

== system Rod_end_v7c/Molla attuatore ==
  X_att : Inport
  V_att : Inport  Port=2
  Pos_out : Inport  Port=3
  Vel_out : Inport  Port=4
  Rot_out : Inport  Port=5
  Rot_matrix_out : Inport  Port=6
  Alpha_p : Inport  Port=7
  Alpha_p_d : Inport  Port=8
  Linear component : Subsystem
  Rotational  component : Subsystem
  F_ma : Outport
  M_ext : Outport  Port=2
  wires:
  Rot_matrix_out/1 -> Rotational  component/1(Rot_matrix_out)
  Linear component/1(F_ma) -> F_ma/1
  V_att/1 -> Linear component/2(V_att)
  Vel_out/1 -> Linear component/4(Vel_out)
  X_att/1 -> Linear component/1(X_att)
  Pos_out/1 -> Linear component/3(Pos_out)
  Rotational  component/1(M_ext) -> M_ext/1
  Alpha_p/1 -> Rotational  component/2(Alpha_p)
  Rot_out/1 -> Rotational  component/3(Rot_out)
  Alpha_p_d/1 -> Rotational  component/4(Alpha_p_d)

== system Rod_end_v7c/Molla superficie ==
  Pos_in : Inport
  Vel_in : Inport  Port=2
  X_sup : Inport  Port=3
  V_sup : Inport  Port=4
  Rot_in : Inport  Port=5
  Rot_matrix_IN : Inport  Port=6
  Theta : Inport  Port=7
  Theta_d : Inport  Port=8
  Linear component : Subsystem
  Rotational component : Subsystem
  F_ms : Outport
  M_ext : Outport  Port=2
  wires:
  Linear component/1(F_ms) -> F_ms/1
  X_sup/1 -> Linear component/3(X_sup)
  Pos_in/1 -> Linear component/1(Pos_in)
  Vel_in/1 -> Linear component/2(Vel_in)
  V_sup/1 -> Linear component/4(V_sup)
  Rotational component/1(M_ext) -> M_ext/1
  Rot_in/1 -> Rotational component/1(Rot_in)
  Rot_matrix_IN/1 -> Rotational component/2(Rot_matrix_IN)
  Theta/1 -> Rotational component/3(Theta)
  Theta_d/1 -> Rotational component/4(Theta_d)

== system Rod_end_v7c/Subsystem2 ==
  F_ma : Inport
  Alpha : Inport  Port=2
  Cos : Trigonometry  Operator=cos
  Demux : Demux  Outputs=3
  Divide : Product  Inputs=*/
  Terminator : Terminator
  Terminator1 : Terminator
  F_att : Outport
  wires:
  F_ma/1 -> Demux/1
  Demux/1 -> Divide/1
  Alpha/1 -> Cos/1
  Cos/1 -> Divide/2
  Divide/1 -> F_att/1
  Demux/3 -> Terminator/1
  Demux/2 -> Terminator1/1

== system Rod_end_v7c/Anello Esterno/Magnitude ==
  vect : Inport
  Add2 : Sum  Inputs=+++
  Demux : Demux  Outputs=3
  Math Function : Math  Operator=square  SignedPower=on
  Math Function1 : Math  Operator=square  SignedPower=on
  Math Function2 : Math  Operator=square  SignedPower=on
  Sqrt : Sqrt
  mag : Outport  VectorParamsAs1DForOutWhenUnconnected=off
  wires:
  vect/1 -> Demux/1
  Add2/1 -> Sqrt/1
  Math Function2/1 -> Add2/3
  Demux/1 -> Math Function/1
  Math Function1/1 -> Add2/2
  Math Function/1 -> Add2/1
  Demux/3 -> Math Function2/1
  Demux/2 -> Math Function1/1
  Sqrt/1 -> mag/1

== system Rod_end_v7c/Anello Esterno/Subsystem ==
  note: phidot
  note: thetadot
  note: psidot
  p q r : Inport
  psi theta phi : Inport  Port=2
  Fcn : Fcn  Expr=u(1)+(u(6)*u(5)/u(8)*u(2))+(u(9)*u(5)/u(8)*u(3))
  Fcn1 : Fcn  Expr=u(9)*u(2)-u(6)*u(3)
  Fcn2 : Fcn  Expr=(u(6)/u(8)*u(2))+(u(9)/u(8)*u(3))
  Mux : Mux  Inputs=3
  Mux1 : Mux  Inputs=3
  Trigonometric Function : Trigonometry
  Trigonometric Function1 : Trigonometry  Operator=cos
  psidot thetadot phidot : Outport
  wires:
  psi theta phi/1 -> Trigonometric Function1/1, Trigonometric Function/1
  p q r/1 -> Mux/1
  Trigonometric Function/1 -> Mux/2
  Trigonometric Function1/1 -> Mux/3
  Mux1/1 -> psidot thetadot phidot/1
  Fcn1/1 -> Mux1/2
  Mux/1 -> Fcn2/1, Fcn/1, Fcn1/1
  Fcn2/1 -> Mux1/1
  Fcn/1 -> Mux1/3

== system Rod_end_v7c/Anello Esterno/Subsystem1 ==
  psi theta phi : Inport
  Create 3x3 Matrix : sharedutil/Create 3x3 Matrix  aMode=aMode
      settings: LibrarySourceBlock=aerolibutil/Create 3x3 Matrix
  Fcn : Fcn  Expr=u(5)*u(4)
  Fcn1 : Fcn  Expr=u(5)*u(1)
  Fcn2 : Fcn  Expr=-u(2)
  Fcn3 : Fcn  Expr=u(3)*u(2)*u(4)-u(6)*u(1)
  Fcn4 : Fcn  Expr=u(3)*u(2)*u(1)+u(6)*u(4)
  Fcn5 : Fcn  Expr=u(3)*u(5)
  Fcn6 : Fcn  Expr=u(6)*u(2)*u(4)+u(3)*u(1)
  Fcn7 : Fcn  Expr=u(6)*u(2)*u(1)-u(3)*u(4)
  Fcn8 : Fcn  Expr=u(6)*u(5)
  Mux : Mux  Inputs=2
  Trigonometric Function : Trigonometry
  Trigonometric Function1 : Trigonometry  Operator=cos
  Rot_matrix : Outport
  wires:
  psi theta phi/1 -> Trigonometric Function/1, Trigonometric Function1/1
  Trigonometric Function/1 -> Mux/1
  Trigonometric Function1/1 -> Mux/2
  Fcn8/1 -> Create 3x3 Matrix/9
  Fcn7/1 -> Create 3x3 Matrix/8
  Fcn6/1 -> Create 3x3 Matrix/7
  Fcn5/1 -> Create 3x3 Matrix/6
  Fcn4/1 -> Create 3x3 Matrix/5
  Fcn3/1 -> Create 3x3 Matrix/4
  Fcn2/1 -> Create 3x3 Matrix/3
  Fcn1/1 -> Create 3x3 Matrix/2
  Fcn/1 -> Create 3x3 Matrix/1
  Mux/1 -> Fcn/1, Fcn1/1, Fcn2/1, Fcn3/1, Fcn8/1, Fcn7/1, Fcn6/1, Fcn5/1, Fcn4/1
  Create 3x3 Matrix/1 -> Rot_matrix/1

== system Rod_end_v7c/Anello Interno/Magnitude ==
  vect : Inport
  Add2 : Sum  Inputs=+++
  Demux : Demux  Outputs=3
  Math Function : Math  Operator=square  SignedPower=on
  Math Function1 : Math  Operator=square  SignedPower=on
  Math Function2 : Math  Operator=square  SignedPower=on
  Sqrt : Sqrt
  mag : Outport  VectorParamsAs1DForOutWhenUnconnected=off
  wires:
  vect/1 -> Demux/1
  Add2/1 -> Sqrt/1
  Math Function2/1 -> Add2/3
  Demux/1 -> Math Function/1
  Math Function1/1 -> Add2/2
  Math Function/1 -> Add2/1
  Demux/3 -> Math Function2/1
  Demux/2 -> Math Function1/1
  Sqrt/1 -> mag/1

== system Rod_end_v7c/Anello Interno/Subsystem ==
  note: phidot
  note: thetadot
  note: psidot
  p q r : Inport
  psi theta phi : Inport  Port=2
  Fcn : Fcn  Expr=u(1)+(u(6)*u(5)/u(8)*u(2))+(u(9)*u(5)/u(8)*u(3))
  Fcn1 : Fcn  Expr=u(9)*u(2)-u(6)*u(3)
  Fcn2 : Fcn  Expr=(u(6)/u(8)*u(2))+(u(9)/u(8)*u(3))
  Mux : Mux  Inputs=3
  Mux1 : Mux  Inputs=3
  Trigonometric Function : Trigonometry
  Trigonometric Function1 : Trigonometry  Operator=cos
  psidot thetadot phidot : Outport
  wires:
  psi theta phi/1 -> Trigonometric Function1/1, Trigonometric Function/1
  p q r/1 -> Mux/1
  Trigonometric Function/1 -> Mux/2
  Trigonometric Function1/1 -> Mux/3
  Mux1/1 -> psidot thetadot phidot/1
  Fcn1/1 -> Mux1/2
  Mux/1 -> Fcn2/1, Fcn/1, Fcn1/1
  Fcn2/1 -> Mux1/1
  Fcn/1 -> Mux1/3

== system Rod_end_v7c/Anello Interno/Subsystem1 ==
  psi theta phi : Inport
  Create 3x3 Matrix : sharedutil/Create 3x3 Matrix  aMode=aMode
      settings: LibrarySourceBlock=aerolibutil/Create 3x3 Matrix
  Fcn : Fcn  Expr=u(5)*u(4)
  Fcn1 : Fcn  Expr=u(5)*u(1)
  Fcn2 : Fcn  Expr=-u(2)
  Fcn3 : Fcn  Expr=u(3)*u(2)*u(4)-u(6)*u(1)
  Fcn4 : Fcn  Expr=u(3)*u(2)*u(1)+u(6)*u(4)
  Fcn5 : Fcn  Expr=u(3)*u(5)
  Fcn6 : Fcn  Expr=u(6)*u(2)*u(4)+u(3)*u(1)
  Fcn7 : Fcn  Expr=u(6)*u(2)*u(1)-u(3)*u(4)
  Fcn8 : Fcn  Expr=u(6)*u(5)
  Mux : Mux  Inputs=2
  Trigonometric Function : Trigonometry
  Trigonometric Function1 : Trigonometry  Operator=cos
  Rot_matrix : Outport
  wires:
  psi theta phi/1 -> Trigonometric Function/1, Trigonometric Function1/1
  Trigonometric Function/1 -> Mux/1
  Trigonometric Function1/1 -> Mux/2
  Fcn8/1 -> Create 3x3 Matrix/9
  Fcn7/1 -> Create 3x3 Matrix/8
  Fcn6/1 -> Create 3x3 Matrix/7
  Fcn5/1 -> Create 3x3 Matrix/6
  Fcn4/1 -> Create 3x3 Matrix/5
  Fcn3/1 -> Create 3x3 Matrix/4
  Fcn2/1 -> Create 3x3 Matrix/3
  Fcn1/1 -> Create 3x3 Matrix/2
  Fcn/1 -> Create 3x3 Matrix/1
  Mux/1 -> Fcn/1, Fcn1/1, Fcn2/1, Fcn3/1, Fcn8/1, Fcn7/1, Fcn6/1, Fcn5/1, Fcn4/1
  Create 3x3 Matrix/1 -> Rot_matrix/1

== system Rod_end_v7c/Attuatore/A//D feedback1 ==
  In1 : Inport
  L_hight[ft]2 : Constant  Value=Del_on
  Product : Product  RndMeth=Zero
  Quantizer : Quantizer  QuantizationInterval=QI_AD
  Quantizer1 : Quantizer  QuantizationInterval=QI_AD
  "Sampler " : ZeroOrderHold  SampleTime=ST_AD
  Sum : Sum  Inputs=|++
  Uniform Random Number1 : UniformRandomNumber  Minimum=-4*2.5757e-006  Maximum=4*2.5757e-006  SampleTime=1
  Out3 : Outport
  wires:
  "Sampler "/1 -> Quantizer/1
  In1/1 -> "Sampler "/1  "F/B_A [m]"
  Uniform Random Number1/1 -> Quantizer1/1
  Quantizer/1 -> Sum/1  "F/B_D [m]"
  Sum/1 -> Out3/1  "F/B_D [m]"
  Product/1 -> Sum/2
  Quantizer1/1 -> Product/1  "Noise A/D"
  L_hight[ft]2/1 -> Product/2

== system Rod_end_v7c/Attuatore/Actuation System ==
  Fa_rod [N] : Inport
  In1 : Inport  Port=2
  A2[m2]1 : Gain  Gain=60000
  Actuator : Subsystem
  Mux1 : Mux  Inputs=2
  Scope : Scope
  Servovalve : Subsystem
  To Workspace1 : ToWorkspace  VariableName=Att_Xdd  SampleTime=-1
  To Workspace2 : ToWorkspace  VariableName=Att_Q1  SampleTime=-1
  To Workspace20 : ToWorkspace  VariableName=Att_P1_P2  SampleTime=-1
  To Workspace3 : ToWorkspace  VariableName=Att_Q2  SampleTime=-1
  imposed shutoff valve external position : Constant  Value=xmax_sb
  x  [m] : Outport
  x_d  [m/s] : Outport  Port=2
  x_dd  [m/s^2] : Outport  Port=3
  Out1 : Outport  Port=4
  wires:
  In1/1 -> Servovalve/2(In1)
  Actuator/2(Out3) -> x  [m]/1
  Actuator/3(Out1) -> x_d  [m/s]/1  "x_d[m/s]"
  Servovalve/1(Out4) -> Mux1/1, To Workspace2/1, Actuator/1(In1)
  Servovalve/2(Out1) -> To Workspace3/1, Actuator/2(In3), Mux1/2
  Actuator/1(Out2) -> Out1/1, To Workspace20/1, Servovalve/1(In2)  "P1;P2[Pa]"
  imposed shutoff valve external position/1 -> Servovalve/3(In3)  "X_shutoff [m]"
  Mux1/1 -> A2[m2]1/1
  A2[m2]1/1 -> Scope/1
  Fa_rod [N]/1 -> Actuator/3(" ")
  Actuator/4(Out5) -> To Workspace1/1, x_dd  [m/s^2]/1  "x_dd[m/s^2]"

== system Rod_end_v7c/Attuatore/Controller Actuator1 ==
  In2 : Inport
  Input : Inport  Port=2
  A2[m2] : Gain  Gain=0.5
  A2[m2]1 : Gain  Gain=0.5
  A2[m2]2 : Gain  Gain=Voltage_com
  A2[m2]3 : Gain  Gain=1/Resistance
  Gain : Gain  Gain=2
  Gain1 : Gain  Gain=0.02
  Gain2 : Gain  Gain=2
  Gain3 : Gain  Gain=0.02
  Integrator : Integrator
  Integrator1 : Integrator
  Mux1 : Mux  Inputs=2
  Null shift : Subsystem  Commented=on
  Scope : Scope
  Step1 : Step  Time=0.3  After=L_c  SampleTime=0
  Subtract : Sum  Inputs=-+
  Subtract1 : Sum  Inputs=-+
  Sum : Sum
  Sum1 : Sum
  Sum2 : Sum  Inputs=|++
  controller error : ManualSwitch
  Out1 : Outport
  Out2 : Outport  Port=2
  wires:
  A2[m2]1/1 -> Mux1/2
  A2[m2]/1 -> Mux1/1
  Input/1 -> Subtract1/2, Subtract/2
  Mux1/1 -> controller error/1  "icom(1,2)[A]"
  controller error/1 -> A2[m2]2/1
  Step1/1 -> controller error/2
  A2[m2]2/1 -> A2[m2]3/1, Out2/1  "Vcom(1,2)[A]"
  A2[m2]3/1 -> Sum2/1, Null shift/1(In2)  "icom(1,2)[A]"
  Null shift/1(Out2) -> Sum2/2, Scope/1
  Sum2/1 -> Out1/1  "icom(1,2)[A]"
  Gain/1 -> Sum/1
  Subtract/1 -> Gain1/1, Gain/1
  Subtract1/1 -> Gain3/1, Gain2/1
  Gain2/1 -> Sum1/1
  Sum1/1 -> A2[m2]1/1
  Sum/1 -> A2[m2]/1
  In2/1 -> Subtract/1, Subtract1/1
  Gain1/1 -> Integrator/1
  Integrator/1 -> Sum/2
  Gain3/1 -> Integrator1/1
  Integrator1/1 -> Sum1/2

== system Rod_end_v7c/Attuatore/Fluid ==
  In1 : Inport
  Mux2 : Mux  Inputs=2
  Product2 : Product  RndMeth=Zero
  tt : Fcn  Expr=(-0.85*u(1)+1015.4)*(1+20/8000)
  tt1 : Fcn  Expr=(1e-6*10^(0.3829*log10(u(1) +51)^4-1.8481*log10(u(1) +51)^3+2.2079*log10(u(1) +51)^2-1.1052*log10(u(1) +51)+2.9544))
  "{ro mu}" : Outport
  tag scope: only_viscosity_var=global
  wires:
  In1/1 -> tt1/1, tt/1
  tt/1 -> Mux2/1, Product2/1  "ro"
  Product2/1 -> Mux2/2, [only_viscosity_var]  "mu"
  tt1/1 -> Product2/2
  Mux2/1 -> "{ro mu}"/1

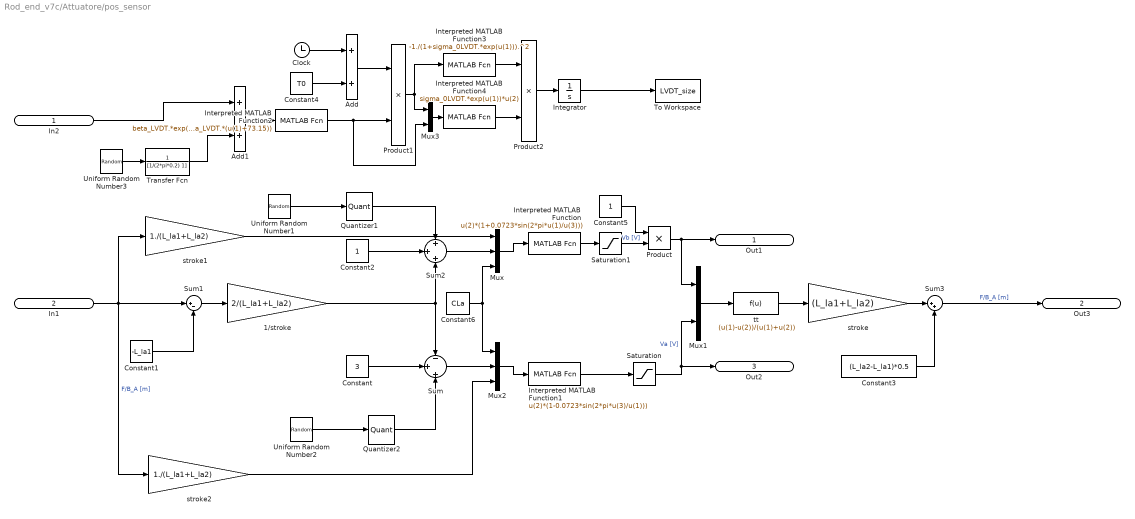
== system Rod_end_v7c/Attuatore/pos_sensor ==
  In2 : Inport
  In1 : Inport  Port=2
  1/stroke : Gain  Gain=2/(L_la1+L_la2)  SaturateOnIntegerOverflow=on  OutDataTypeStr=Inherit: Same as input  ParamDataTypeStr=Inherit: Same as input
  Add : Sum
  Add1 : Sum
  Clock : Clock
  Constant : Constant  Value=3
  Constant1 : Constant  Value=-L_la1
  Constant2 : Constant
  Constant3 : Constant  Value=(L_la2-L_la1)*0.5
  Constant4 : Constant  Value=T0
  Constant5 : Constant
  Constant6 : Constant  Value=CLa
  Integrator : Integrator  InitialCondition=LVDTsize0
  Interpreted MATLAB Function : MATLABFcn  MATLABFcn=u(2)*(1+0.0723*sin(2*pi*u(1)/u(3)))
  Interpreted MATLAB Function1 : MATLABFcn  MATLABFcn=u(2)*(1-0.0723*sin(2*pi*u(3)/u(1)))
  Interpreted MATLAB Function2 : MATLABFcn  MATLABFcn=beta_LVDT.*exp(lambda_LVDT.*(u(1)+73.15))
  Interpreted MATLAB Function3 : MATLABFcn  MATLABFcn=-1./(1+sigma_0LVDT.*exp(u(1))).^2
  Interpreted MATLAB Function4 : MATLABFcn  MATLABFcn=sigma_0LVDT.*exp(u(1))*u(2)
  Mux : Mux  Inputs=3
  Mux1 : Mux  Inputs=2
  Mux2 : Mux  Inputs=3
  Mux3 : Mux  Inputs=2
  Product : Product
  Product1 : Product
  Product2 : Product
  Quantizer1 : Quantizer  QuantizationInterval=4/(2^14)
  Quantizer2 : Quantizer  QuantizationInterval=4/(2^14)
  Saturation : Saturate  UpperLimit=3  LowerLimit=1
  Saturation1 : Saturate  UpperLimit=3  LowerLimit=1
  Sum : Sum  Inputs=-|+|+
  Sum1 : Sum  Inputs=|+-
  Sum2 : Sum  Inputs=+|+|+
  Sum3 : Sum  Inputs=|++
  To Workspace : ToWorkspace  VariableName=LVDT_size  SaveFormat=Structure With Time  SampleTime=-1
  Transfer Fcn : TransferFcn  Denominator=[1/(2*pi*0.2) 1]
  Uniform Random Number1 : UniformRandomNumber  Minimum=-0.02*2  Maximum=0.02*2
  Uniform Random Number2 : UniformRandomNumber  Minimum=-0.02*2  Maximum=0.02*2
  Uniform Random Number3 : UniformRandomNumber  Minimum=-20  Maximum=20  Seed=rand(1)  SampleTime=10
  stroke : Gain  Gain=(L_la1+L_la2)  SaturateOnIntegerOverflow=on  OutDataTypeStr=Inherit: Same as input  ParamDataTypeStr=Inherit: Same as input
  stroke1 : Gain  Gain=1./(L_la1+L_la2)  SaturateOnIntegerOverflow=on  OutDataTypeStr=Inherit: Same as input  ParamDataTypeStr=Inherit: Same as input
  stroke2 : Gain  Gain=1./(L_la1+L_la2)  SaturateOnIntegerOverflow=on  OutDataTypeStr=Inherit: Same as input  ParamDataTypeStr=Inherit: Same as input
  tt : Fcn  Expr=(u(1)-u(2))/(u(1)+u(2))
  Out1 : Outport
  Out3 : Outport  Port=2
  Out2 : Outport  Port=3
  wires:
  In1/1 -> stroke2/1, stroke1/1, Sum1/1  "F/B_A [m]"
  Constant1/1 -> Sum1/2
  Sum1/1 -> 1/stroke/1
  Constant/1 -> Sum/2
  1/stroke/1 -> Sum/1, Sum2/3
  Constant2/1 -> Sum2/2
  Mux1/1 -> tt/1
  tt/1 -> stroke/1
  Sum3/1 -> Out3/1  "F/B_A [m]"
  Constant3/1 -> Sum3/2
  stroke/1 -> Sum3/1
  Uniform Random Number1/1 -> Quantizer1/1
  Uniform Random Number2/1 -> Quantizer2/1
  Quantizer1/1 -> Sum2/1
  Quantizer2/1 -> Sum/3
  Saturation/1 -> Out2/1, Mux1/2  "Va [V]"
  Sum2/1 -> Mux/2
  stroke1/1 -> Mux/1
  Interpreted MATLAB Function/1 -> Saturation1/1
  Mux/1 -> Interpreted MATLAB Function/1
  Mux2/1 -> Interpreted MATLAB Function1/1
  Interpreted MATLAB Function1/1 -> Saturation/1
  Product/1 -> Mux1/1, Out1/1
  Saturation1/1 -> Product/2  "Vb [V]"
  Constant4/1 -> Add/2
  Clock/1 -> Add/1
  Interpreted MATLAB Function2/1 -> Mux3/2, Product1/2
  Add/1 -> Product1/1
  Product1/1 -> Mux3/1, Interpreted MATLAB Function3/1
  Add1/1 -> Interpreted MATLAB Function2/1
  In2/1 -> Add1/1
  Uniform Random Number3/1 -> Transfer Fcn/1
  Transfer Fcn/1 -> Add1/2
  Interpreted MATLAB Function3/1 -> Product2/1
  Interpreted MATLAB Function4/1 -> Product2/2
  Product2/1 -> Integrator/1
  Integrator/1 -> To Workspace/1
  Mux3/1 -> Interpreted MATLAB Function4/1
  Constant5/1 -> Product/1
  stroke2/1 -> Mux2/3
  Sum/1 -> Mux2/2
  Constant6/1 -> Mux2/1, Mux/3

== system Rod_end_v7c/Contatto/Damping component ==
  note: c'è un errore qua secondo me
  note: Fdamp
  note: Delta_d
  Delta_n : Inport
  F_spring : Inport  Port=2
  VelIN : Inport  Port=3
  VelOUT : Inport  Port=4
  Fc : Inport  Port=5
  Add2 : Sum  Inputs=+-
  Constant : Constant  Value=1e2
  Magnitude2 : Subsystem
  Min : MinMax  Inputs=2
  Product : Product
  Subsystem1 : Subsystem
  To Workspace2 : ToWorkspace  VariableName=simout  SampleTime=-1
  F_damp : Outport
  wires:
  Min/1 -> F_damp/1
  Product/1 -> Min/2
  Magnitude2/1(mag) -> Subsystem1/2(Delta_d), Product/1
  F_spring/1 -> Min/1
  VelIN/1 -> Add2/1
  Add2/1 -> Magnitude2/1(vect)
  VelOUT/1 -> Add2/2
  Subsystem1/1(D) -> To Workspace2/1
  Delta_n/1 -> Subsystem1/1(Delta_n)
  Fc/1 -> Subsystem1/3(Fc)
  Constant/1 -> Product/2

== system Rod_end_v7c/Contatto/Stiffness component ==
  Delta : Inport
  Constant6 : Constant  Value=3/2
  Constant7 : Constant  Value=k
  Math Function3 : Math  Operator=pow
  Product8 : Product
  F_spring : Outport
  Delta_n : Outport  Port=2
  wires:
  Constant7/1 -> Product8/2
  Constant6/1 -> Math Function3/2
  Math Function3/1 -> Delta_n/1, Product8/1
  Delta/1 -> Math Function3/1
  Product8/1 -> F_spring/1

== system Rod_end_v7c/Contatto/Subsystem ==
  note: Versore eccentricità
  note: Clearance
  note: Delta
  PosIN : Inport
  PosOUT : Inport  Port=2
  Add : Sum  Inputs=+-
  Add1 : Sum  Inputs=+-
  Add6 : Sum  Inputs=+-
  Constant3 : Constant  Value=R_out
  Constant5 : Constant  Value=R_in
  Constant8 : Constant
  Magnitude : Subsystem
  Product1 : Product  Inputs=*/
  Reshape2 : Reshape  OutputDimensionality=Column vector (2-D)
  Switch1 : Switch  Criteria=u2 ~= 0  SaturateOnIntegerOverflow=off  InputSameDT=off
  e : Outport
  Dir_e : Outport  Port=2
  Delta : Outport  Port=3
  wires:
  Switch1/1 -> Product1/2
  Add/1 -> Magnitude/1(vect), Product1/1
  Constant8/1 -> Switch1/3
  Add6/1 -> Add1/2
  Magnitude/1(mag) -> Add1/1, Switch1/1, Switch1/2, e/1
  Constant5/1 -> Add6/2
  Reshape2/1 -> Dir_e/1
  PosOUT/1 -> Add/2
  Product1/1 -> Reshape2/1
  PosIN/1 -> Add/1
  Constant3/1 -> Add6/1
  Add1/1 -> Delta/1

== system Rod_end_v7c/Contatto/Subsystem1 ==
  note: mu
  Fc : Inport
  V_IN : Inport  Port=2
  V_OUT : Inport  Port=3
  1-D Lookup Table : Lookup_n-D  NumberOfTableDimensions=1  BreakpointsForDimension1=v_rel  Table=muu  InternalRulePriority=Speed  RndMeth=Simplest
  Add9 : Sum  Inputs=+-
  Constant9 : Constant
  Divide : Product  Inputs=*/
  Gain1 : Gain  Gain=-1
  Magnitude1 : Subsystem
  Product6 : Product
  Product7 : Product
  Scope3 : Scope
  Switch2 : Switch  Criteria=u2 ~= 0  SaturateOnIntegerOverflow=off  InputSameDT=off
  Fattr : Outport
  Vrel : Outport  Port=2
  wires:
  V_OUT/1 -> Add9/2
  Switch2/1 -> Divide/2
  Product6/1 -> Product7/2
  Constant9/1 -> Switch2/3
  Add9/1 -> Vrel/1, Divide/1, Magnitude1/1(vect)
  Fc/1 -> Product6/1
  Magnitude1/1(mag) -> Switch2/2, Switch2/1, 1-D Lookup Table/1
  Gain1/1 -> Scope3/1, Product7/1
  Product7/1 -> Fattr/1
  V_IN/1 -> Add9/1
  Divide/1 -> Gain1/1
  1-D Lookup Table/1 -> Product6/2

== system Rod_end_v7c/Contatto/Vel_contatto_IN ==
  note: Vel normale al contatto
  note: Raggio_IN
  note: Velocità di trascinamento
  note: Vel tangenziale al contatto
  note: Raggio
      | (Vettore)
  Dir_e : Inport
  Vel_IN : Inport  Port=2
  RotIN : Inport  Port=3
  Add4 : Sum
  Add5 : Sum  Inputs=-+
  Constant2 : Constant  Value=R_in
  Cross Product3 : matrix_library/Cross Product
  Dot Product : DotProduct  OutDataTypeStr=Inherit: Inherit via internal rule
  Gain1 : Gain  Commented=through  Gain=0
  Gain12 : Gain  Commented=through  Gain=0
  Product10 : Product  Multiplication=Matrix(*)
  Product5 : Product  Multiplication=Matrix(*)
  Vel_tang_IN : Outport
  Raggio_IN : Outport  Port=2
  wires:
  Constant2/1 -> Product10/2
  Add5/1 -> Vel_tang_IN/1
  Dot Product/1 -> Product5/2
  Vel_IN/1 -> Gain12/1
  Dir_e/1 -> Product5/1, Dot Product/1, Product10/1
  RotIN/1 -> Cross Product3/1
  Product5/1 -> Add5/1
  Product10/1 -> Raggio_IN/1, Cross Product3/2
  Add4/1 -> Add5/2, Dot Product/2
  Cross Product3/1 -> Gain1/1
  Gain12/1 -> Add4/1
  Gain1/1 -> Add4/2

== system Rod_end_v7c/Contatto/Vel_contatto_OUT ==
  Dir_e : Inport
  Vel_OUT : Inport  Port=2
  RotOUT : Inport  Port=3
  Add7 : Sum
  Add8 : Sum  Inputs=-+
  Constant10 : Constant  Value=R_out
  Cross Product2 : matrix_library/Cross Product
  Dot Product1 : DotProduct  OutDataTypeStr=Inherit: Inherit via internal rule
  Gain1 : Gain  Commented=through  Gain=0
  Gain12 : Gain  Commented=through  Gain=0
  Product4 : Product  Multiplication=Matrix(*)
  Product9 : Product  Multiplication=Matrix(*)
  Vel_tang_OUT : Outport
  Raggio_OUT : Outport  Port=2
  wires:
  Vel_OUT/1 -> Gain12/1
  Dot Product1/1 -> Product9/2
  Dir_e/1 -> Product9/1, Dot Product1/1, Product4/1
  Cross Product2/1 -> Gain1/1
  Product9/1 -> Add8/1
  Add7/1 -> Add8/2, Dot Product1/2
  Add8/1 -> Vel_tang_OUT/1
  Constant10/1 -> Product4/2
  RotOUT/1 -> Cross Product2/1
  Gain12/1 -> Add7/1
  Gain1/1 -> Add7/2
  Product4/1 -> Cross Product2/2, Raggio_OUT/1
